simulink model "SistemaTotal"  (R2014a)
settings: Solver=ode45  SolverMode=SingleTasking  StartTime=0.0  StopTime=10000  RelTol=1e-3
values from neighbouring files (symbols this model uses):
  G = 0    [Variaveis.mat]
  M = 0.95    [Variaveis.mat]
  T = 1    [Variaveis.mat]
settings Model: CovSFcnEnable=on  Creator=Afonso  LastModifiedBy=pedropinto
settings DataIOCC: SignalLoggingSaveFormat=ModelDataLogs
settings OptimizationCC: BlockReduction=off  BooleanDataType=off  SimCompilerOptimization=off
settings DebuggingCC: SaveWithParameterizedLinksMsg=none  UnderspecifiedInitializationDetection=Classic  SignalResolutionControl=TryResolveAllWithWarning  SolverPrmCheckMsg=none  MultiTaskDSMMsg=warning  MultiTaskCondExecSysMsg=none  FrameProcessingCompatibilityMsg=error  StrictBusMsg=None
settings HardwareCC: TargetUnknown=on
settings RTWCC: RTWCompilerOptimization=off

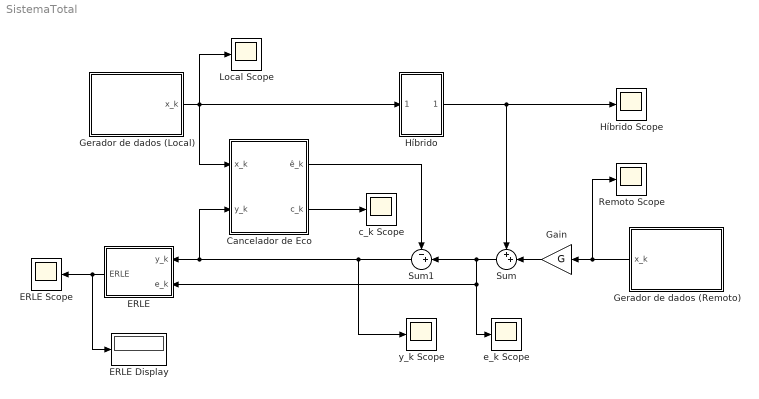
== system SistemaTotal ==
  Cancelador de Eco : Subsystem
  ERLE : Subsystem
  ERLE Display : Display
  ERLE Scope : Scope
      settings: TimeRange=1400  YMin=-61.5  YMax=-58.25  SaveName=ERLE
  Gain : Gain  Gain=G
  Gerador de dados (Local) : Subsystem
  Gerador de dados (Remoto) : Subsystem
  Híbrido : Subsystem
  Híbrido Scope : Scope
      settings: SaveName=Hibrido
  Local Scope : Scope
      settings: SaveName=Local
  Remoto Scope : Scope
      settings: SaveName=Remoto
  Sum : Sum  Inputs=++|
  Sum1 : Sum  Inputs=-+|
  "c_k Scope " : Scope
      settings: SaveName=Coeficientes
  e_k Scope : Scope
      settings: SaveName=Eco
  y_k Scope : Scope
      settings: SaveName=Erro
  wires:
  Gerador de dados (Local)/1(x_k) -> Cancelador de Eco/1(x_k), Híbrido/1(x_k), Local Scope/1
  Gerador de dados (Remoto)/1(x_k) -> Remoto Scope/1, Gain/1
  Gain/1 -> Sum/2
  Híbrido/1(Out1) -> Híbrido Scope/1, Sum/1
  Cancelador de Eco/1(ê_k) -> Sum1/1
  ERLE/1(ERLE) -> ERLE Display/1, ERLE Scope/1
  Sum/1 -> ERLE/2(e_k), e_k Scope/1, Sum1/2
  Sum1/1 -> y_k Scope/1, Cancelador de Eco/2(y_k), ERLE/1(y_k)
  Cancelador de Eco/2(c_k) -> "c_k Scope "/1

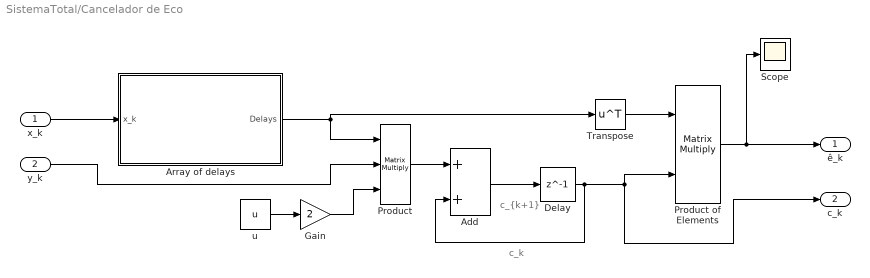
== system SistemaTotal/Cancelador de Eco ==
  note: c_k
  note: c_{k+1}
  x_k : Inport
  y_k : Inport  Port=2
  Add : Sum
  Array of delays : Subsystem
  Delay : Delay  DelayLength=1  SampleTime=T
  Gain : Gain  Gain=2
  Product : Product  Inputs=3  Multiplication=Matrix(*)
  Product of Elements : Product  Inputs=**  Multiplication=Matrix(*)
  Scope : Scope
  Transpose : Math  Operator=transpose  SaturateOnIntegerOverflow=on
  u : Constant  Value=u  SampleTime=T
  ê_k : Outport
  c_k : Outport  Port=2
  wires:
  y_k/1 -> Product/2
  u/1 -> Gain/1
  Gain/1 -> Product/3
  x_k/1 -> Array of delays/1(x_k)
  Product/1 -> Add/1
  Product of Elements/1 -> ê_k/1, Scope/1
  Add/1 -> Delay/1
  Delay/1 -> c_k/1, Product of Elements/2, Add/2
  Transpose/1 -> Product of Elements/1
  Array of delays/1(Delays) -> Product/1, Transpose/1

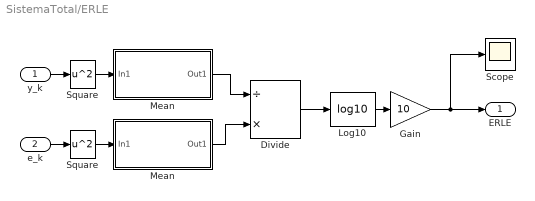
== system SistemaTotal/ERLE ==
  y_k : Inport
  e_k : Inport  Port=2
  Divide : Product  Inputs=/*
  Gain : Gain  Gain=10
  Log10 : Math  Operator=log10  SaturateOnIntegerOverflow=on
  Mean : Subsystem
  "Mean " : Subsystem
  Scope : Scope
  Square : Math  Operator=square  SaturateOnIntegerOverflow=on
  "Square " : Math  Operator=square  SaturateOnIntegerOverflow=on
  ERLE : Outport
  wires:
  e_k/1 -> "Square "/1
  y_k/1 -> Square/1
  "Square "/1 -> "Mean "/1(In1)
  "Mean "/1(Out1) -> Divide/2
  Log10/1 -> Gain/1
  Divide/1 -> Log10/1
  Gain/1 -> ERLE/1, Scope/1
  Mean/1(Out1) -> Divide/1
  Square/1 -> Mean/1(In1)

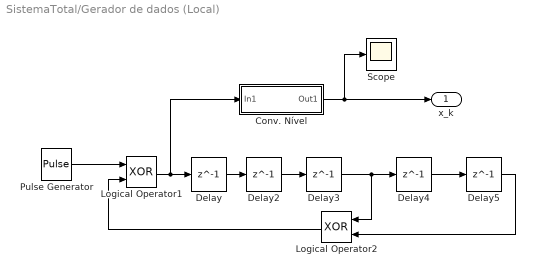
== system SistemaTotal/Gerador de dados (Local) ==
  Conv. Nível : Subsystem
  Delay : Delay  DelayLength=1  SampleTime=T
  Delay{2..5} (4 alike) : Delay  DelayLength=1
  Logical Operator1 : Logic  Operator=XOR  AllPortsSameDT=off  OutDataTypeStr=boolean
  Logical Operator2 : Logic  Operator=XOR  AllPortsSameDT=off  OutDataTypeStr=boolean
  Pulse Generator : DiscretePulseGenerator  PulseType=Time based  Period=2*T  PulseWidth=50
  Scope : Scope
      settings: YMin=-1.5  YMax=1.5
  x_k : Outport
  wires:
  Delay2/1 -> Delay3/1
  Delay/1 -> Delay2/1
  Delay4/1 -> Delay5/1
  Delay3/1 -> Logical Operator2/1, Delay4/1
  Logical Operator2/1 -> Logical Operator1/2
  Delay5/1 -> Logical Operator2/2
  Logical Operator1/1 -> Conv. Nível/1(In1), Delay/1
  Conv. Nível/1(Out1) -> x_k/1, Scope/1
  Pulse Generator/1 -> Logical Operator1/1

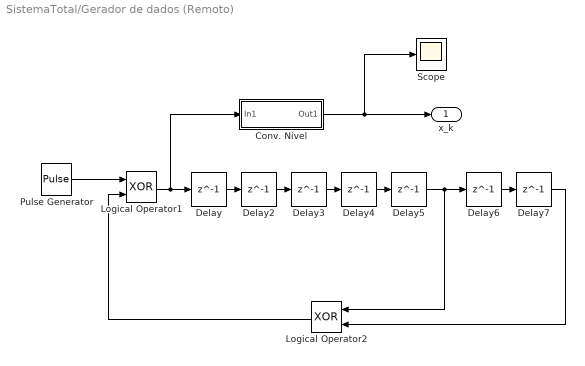
== system SistemaTotal/Gerador de dados (Remoto) ==
  Conv. Nível : Subsystem
  Delay : Delay  DelayLength=1  SampleTime=T
  Delay{2..7} (6 alike) : Delay  DelayLength=1
  Logical Operator1 : Logic  Operator=XOR  AllPortsSameDT=off  OutDataTypeStr=boolean
  Logical Operator2 : Logic  Operator=XOR  AllPortsSameDT=off  OutDataTypeStr=boolean
  Pulse Generator : DiscretePulseGenerator  PulseType=Time based  Period=2*T  PulseWidth=50
  Scope : Scope
  x_k : Outport
  wires:
  Logical Operator1/1 -> Conv. Nível/1(In1), Delay/1
  Delay4/1 -> Delay5/1
  Conv. Nível/1(Out1) -> x_k/1, Scope/1
  Delay7/1 -> Logical Operator2/2
  Pulse Generator/1 -> Logical Operator1/1
  Logical Operator2/1 -> Logical Operator1/2
  Delay6/1 -> Delay7/1
  Delay5/1 -> Delay6/1, Logical Operator2/1
  Delay2/1 -> Delay3/1
  Delay/1 -> Delay2/1
  Delay3/1 -> Delay4/1

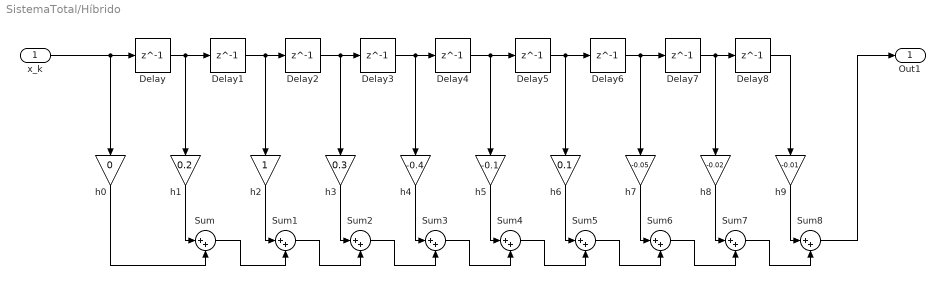
== system SistemaTotal/Híbrido ==
  x_k : Inport
  Delay{,1..8} (9 alike) : Delay  DelayLength=1  SampleTime=T
  Sum{,1..8} (9 alike) : Sum  Inputs=|++
  h0 : Gain  Gain=0
  h1 : Gain  Gain=0.2
  h2 : Gain
  h3 : Gain  Gain=0.3
  h4 : Gain  Gain=-0.4
  h5 : Gain  Gain=-0.1
  h6 : Gain  Gain=0.1
  h7 : Gain  Gain=-0.05
  h8 : Gain  Gain=-0.02
  h9 : Gain  Gain=-0.01
  Out1 : Outport
  wires:
  Sum5/1 -> Sum6/2
  Sum1/1 -> Sum2/2
  Sum6/1 -> Sum7/2
  h9/1 -> Sum8/1
  Sum4/1 -> Sum5/2
  Sum7/1 -> Sum8/2
  Sum3/1 -> Sum4/2
  Sum8/1 -> Out1/1
  Sum2/1 -> Sum3/2
  h7/1 -> Sum6/1
  h8/1 -> Sum7/1
  Delay1/1 -> Delay2/1, h2/1
  Delay/1 -> Delay1/1, h1/1
  Delay2/1 -> Delay3/1, h3/1
  Delay3/1 -> Delay4/1, h4/1
  Delay4/1 -> Delay5/1, h5/1
  Delay6/1 -> Delay7/1, h7/1
  Sum/1 -> Sum1/2
  h2/1 -> Sum1/1
  Delay8/1 -> h9/1
  h1/1 -> Sum/1
  Delay7/1 -> Delay8/1, h8/1
  x_k/1 -> Delay/1, h0/1
  h0/1 -> Sum/2
  h4/1 -> Sum3/1
  h5/1 -> Sum4/1
  Delay5/1 -> Delay6/1, h6/1
  h3/1 -> Sum2/1
  h6/1 -> Sum5/1

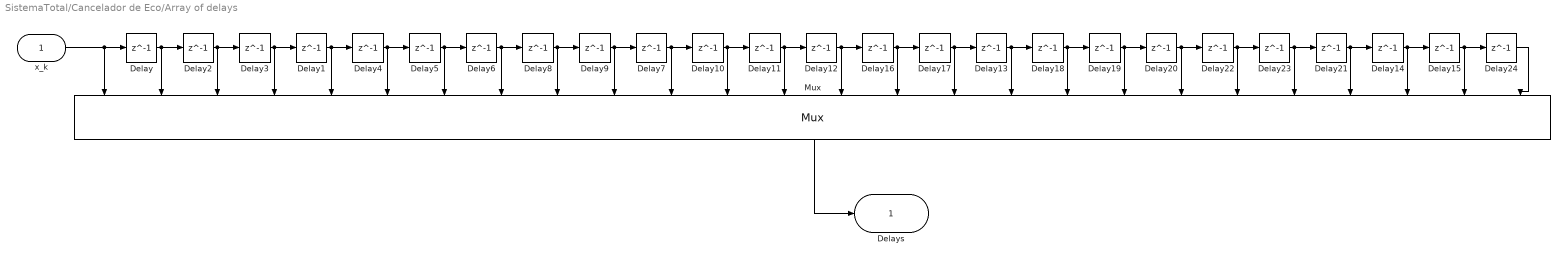
== system SistemaTotal/Cancelador de Eco/Array of delays ==
  x_k : Inport
  Delay : Delay  DelayLength=1  SampleTime=T
  Delay{1..24} (24 alike) : Delay  DelayLength=1
  Mux : Mux  Inputs=26
      settings: DisplayOption=signals
  Delays : Outport
  wires:
  Delay/1 -> Delay2/1, Mux/2
  Delay2/1 -> Mux/3, Delay3/1
  Delay11/1 -> Mux/13, Delay12/1
  Delay24/1 -> Mux/26
  Delay19/1 -> Delay20/1, Mux/19
  x_k/1 -> Delay/1, Mux/1
  Mux/1 -> Delays/1
  Delay15/1 -> Delay24/1, Mux/25
  Delay4/1 -> Mux/6, Delay5/1
  Delay1/1 -> Mux/5, Delay4/1
  Delay5/1 -> Mux/7, Delay6/1
  Delay12/1 -> Mux/14, Delay16/1
  Delay18/1 -> Mux/18, Delay19/1
  Delay16/1 -> Mux/15, Delay17/1
  Delay23/1 -> Delay21/1, Mux/22
  Delay17/1 -> Mux/16, Delay13/1
  Delay22/1 -> Delay23/1, Mux/21
  Delay14/1 -> Delay15/1, Mux/24
  Delay20/1 -> Delay22/1, Mux/20
  Delay13/1 -> Mux/17, Delay18/1
  Delay21/1 -> Delay14/1, Mux/23
  Delay8/1 -> Mux/9, Delay9/1
  Delay6/1 -> Mux/8, Delay8/1
  Delay10/1 -> Delay11/1, Mux/12
  Delay9/1 -> Delay7/1, Mux/10
  Delay7/1 -> Mux/11, Delay10/1
  Delay3/1 -> Mux/4, Delay1/1

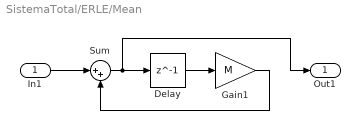
== system SistemaTotal/ERLE/Mean ==
  In1 : Inport
  Delay : Delay  DelayLength=1  SampleTime=T
  Gain1 : Gain  Gain=M
  Sum : Sum  Inputs=|++
  Out1 : Outport
  wires:
  Delay/1 -> Gain1/1
  Gain1/1 -> Sum/2
  In1/1 -> Sum/1
  Sum/1 -> Out1/1, Delay/1

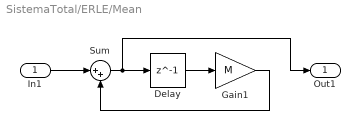
== system SistemaTotal/ERLE/Mean  ==
  In1 : Inport
  Delay : Delay  DelayLength=1  SampleTime=T
  Gain1 : Gain  Gain=M
  Sum : Sum  Inputs=|++
  Out1 : Outport
  wires:
  Delay/1 -> Gain1/1
  Gain1/1 -> Sum/2
  In1/1 -> Sum/1
  Sum/1 -> Out1/1, Delay/1

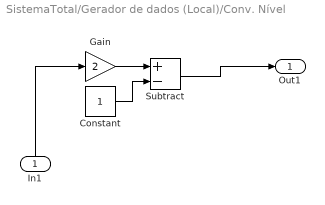
== system SistemaTotal/Gerador de dados (Local)/Conv. Nível ==
  In1 : Inport
  Constant : Constant
  Gain : Gain  Gain=2
  Subtract : Sum  Inputs=+-
  Out1 : Outport
  wires:
  In1/1 -> Gain/1
  Constant/1 -> Subtract/2
  Gain/1 -> Subtract/1
  Subtract/1 -> Out1/1

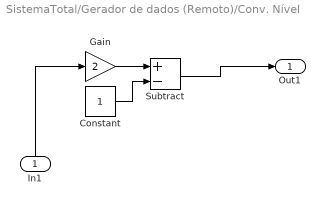
== system SistemaTotal/Gerador de dados (Remoto)/Conv. Nível ==
  In1 : Inport
  Constant : Constant
  Gain : Gain  Gain=2
  Subtract : Sum  Inputs=+-
  Out1 : Outport
  wires:
  In1/1 -> Gain/1
  Constant/1 -> Subtract/2
  Gain/1 -> Subtract/1
  Subtract/1 -> Out1/1
